simulink model "flatsat_data_send_2018"  (R2018b)
settings: Solver=VariableStepAuto  StartTime=0.0  StopTime=Inf  RelTol=1e-3
values from neighbouring files (symbols this model uses):
  bias_sun_detection = 50    [flatsat_data_send_init.m]
  magnitude_gyro = 250    [flatsat_data_send_init.m]
  magnitude_mag = 100    [flatsat_data_send_init.m]
  magnitude_phd = 100    [flatsat_data_send_init.m]
  magnitude_sun_angle = 60    [flatsat_data_send_init.m]
  magnitude_sun_detection = 50    [flatsat_data_send_init.m]
  t_receive_gyro = t_send_gyro    (= 0.04)    [flatsat_data_send_init.m]
  t_receive_sun = t_send_sun    (= 0.02)    [flatsat_data_send_init.m]
  t_send_gyro = 1/25    (= 0.04)    [flatsat_data_send_init.m]
  t_send_mag = 1/15    (= 0.0666666666667)    [flatsat_data_send_init.m]
  t_send_phd = 0.061    [flatsat_data_send_init.m]
  t_send_sun = 0.02    [flatsat_data_send_init.m]
undefined symbols (not defined in the file or in its folder): serial, t_receive
libraries: instrumentlib x12
settings Model: EnablePacing=on  Creator=Alex Zhen  LastModifiedBy=Alex Zhen
settings DataIOCC: ReturnWorkspaceOutputs=on

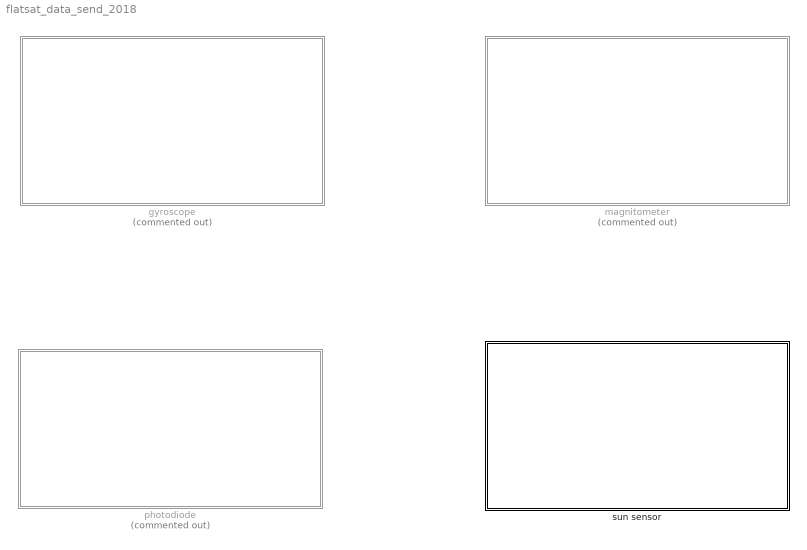
== system flatsat_data_send_2018 ==
  gyroscope : Subsystem  Commented=on
  magnitometer : Subsystem  Commented=on
  photodiode : Subsystem  Commented=on
  sun sensor : Subsystem

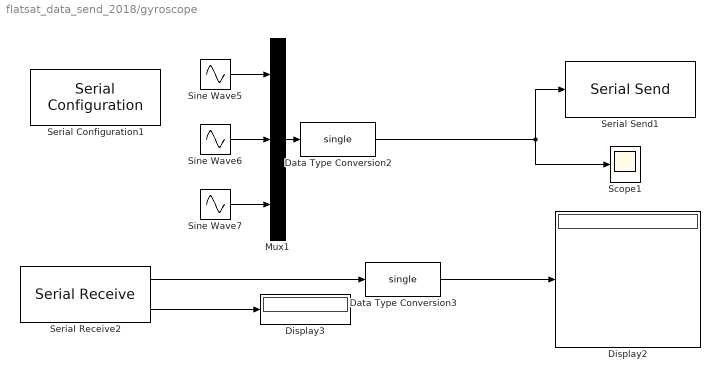
== system flatsat_data_send_2018/gyroscope ==
  Data Type Conversion2 : DataTypeConversion  OutDataTypeStr=single
  Data Type Conversion3 : DataTypeConversion  OutDataTypeStr=single
  Display2 : Display
  Display3 : Display
  Mux1 : Mux  Inputs=3
  Scope1 : Scope
  Serial Configuration1 : instrumentlib/Serial Configuration  Priority=-200000  ComPortMenu=COM5  ComPort=COM5  ObjConstructor=serial('COM5');  BaudRate=115200  DataBits=8  Parity=none  StopBits=1  FlowControl=none  Timeout=10  ByteOrder=LittleEndian
  Serial Receive2 : instrumentlib/Serial Receive  ComPortMenu=COM5  ComPort=COM5  ObjConstructor=serial('COM5');  Terminator=<none>  DataSize="[3  1]"  DataType=single  EnableBlockingMode=off  ActionDataUnavailable=Output last received value  CustomValue=0  SampleTime=t_receive_gyro
  Serial Send1 : instrumentlib/Serial Send  ComPortMenu=COM5  ComPort=COM5  ObjConstructor=serial('COM5');  Terminator=<none>  EnableBlockingMode=off
  Sine Wave5 : Sin  Amplitude=magnitude_gyro  Frequency=pi/5  SampleTime=t_send_gyro
  Sine Wave6 : Sin  Amplitude=magnitude_gyro  Frequency=pi/5  Phase=1  SampleTime=t_send_gyro
  Sine Wave7 : Sin  Amplitude=magnitude_gyro  Frequency=pi/5  Phase=2  SampleTime=t_send_gyro
  wires:
  Data Type Conversion2/1 -> Serial Send1/1, Scope1/1
  Data Type Conversion3/1 -> Display2/1
  Sine Wave5/1 -> Mux1/1
  Serial Receive2/1 -> Data Type Conversion3/1
  Sine Wave6/1 -> Mux1/2
  Sine Wave7/1 -> Mux1/3
  Mux1/1 -> Data Type Conversion2/1
  Serial Receive2/2 -> Display3/1

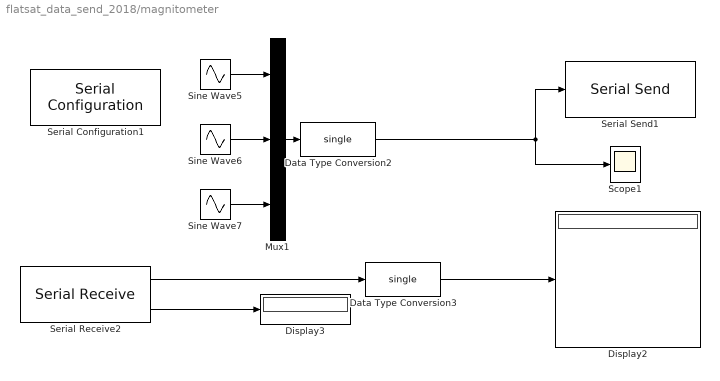
== system flatsat_data_send_2018/magnitometer ==
  Data Type Conversion2 : DataTypeConversion  OutDataTypeStr=single
  Data Type Conversion3 : DataTypeConversion  OutDataTypeStr=single
  Display2 : Display
  Display3 : Display
  Mux1 : Mux  Inputs=3
  Scope1 : Scope
  Serial Configuration1 : instrumentlib/Serial Configuration  Priority=-200000  ComPortMenu=COM5  ComPort=COM5  ObjConstructor=serial('COM5');  BaudRate=115200  DataBits=8  Parity=none  StopBits=1  FlowControl=none  Timeout=10  ByteOrder=LittleEndian
  Serial Receive2 : instrumentlib/Serial Receive  ComPortMenu=COM5  ComPort=COM5  ObjConstructor=serial('COM5');  Terminator=<none>  DataSize="[3  1]"  DataType=single  EnableBlockingMode=off  ActionDataUnavailable=Output last received value  CustomValue=0  SampleTime=t_receive_gyro
  Serial Send1 : instrumentlib/Serial Send  ComPortMenu=COM5  ComPort=COM5  ObjConstructor=serial('COM5');  Terminator=<none>  EnableBlockingMode=off
  Sine Wave5 : Sin  Amplitude=magnitude_mag  Frequency=pi/5  SampleTime=t_send_mag
  Sine Wave6 : Sin  Amplitude=magnitude_mag  Frequency=pi/5  Phase=1  SampleTime=t_send_mag
  Sine Wave7 : Sin  Amplitude=magnitude_mag  Frequency=pi/5  Phase=2  SampleTime=t_send_mag
  wires:
  Data Type Conversion2/1 -> Serial Send1/1, Scope1/1
  Data Type Conversion3/1 -> Display2/1
  Sine Wave5/1 -> Mux1/1
  Serial Receive2/1 -> Data Type Conversion3/1
  Sine Wave6/1 -> Mux1/2
  Sine Wave7/1 -> Mux1/3
  Mux1/1 -> Data Type Conversion2/1
  Serial Receive2/2 -> Display3/1

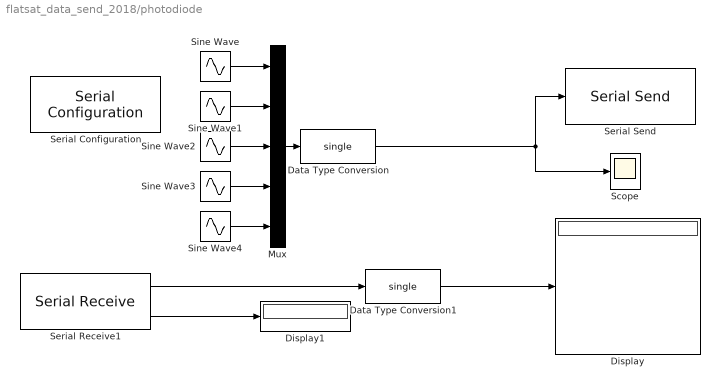
== system flatsat_data_send_2018/photodiode ==
  Data Type Conversion : DataTypeConversion  OutDataTypeStr=single
  Data Type Conversion1 : DataTypeConversion  OutDataTypeStr=single
  Display : Display
  Display1 : Display
  Mux : Mux  Inputs=5
  Scope : Scope
  Serial Configuration : instrumentlib/Serial Configuration  Priority=-200000  ComPortMenu=COM5  ComPort=COM5  ObjConstructor=serial('COM5');  BaudRate=115200  DataBits=8  Parity=none  StopBits=1  FlowControl=none  Timeout=10  ByteOrder=LittleEndian
  Serial Receive1 : instrumentlib/Serial Receive  ComPortMenu=COM5  ComPort=COM5  ObjConstructor=serial('COM5');  Terminator=<none>  DataSize="[5  1]"  DataType=single  EnableBlockingMode=off  ActionDataUnavailable=Output last received value  CustomValue=0  SampleTime=t_receive
  Serial Send : instrumentlib/Serial Send  ComPortMenu=COM5  ComPort=COM5  ObjConstructor=serial('COM5');  Terminator=<none>  EnableBlockingMode=off
  Sine Wave : Sin  Amplitude=magnitude_phd  Frequency=pi/5  SampleTime=t_send_phd
  Sine Wave1 : Sin  Amplitude=250  Frequency=pi/5  Phase=1  SampleTime=t_send_phd
  Sine Wave2 : Sin  Amplitude=magnitude_phd  Frequency=pi/5  Phase=2  SampleTime=t_send_phd
  Sine Wave3 : Sin  Amplitude=magnitude_phd  Frequency=pi/5  Phase=3  SampleTime=t_send_phd
  Sine Wave4 : Sin  Amplitude=magnitude_phd  Frequency=pi/5  Phase=4  SampleTime=t_send_phd
  wires:
  Sine Wave1/1 -> Mux/2
  Data Type Conversion/1 -> Serial Send/1, Scope/1
  Serial Receive1/2 -> Display1/1
  Data Type Conversion1/1 -> Display/1
  Sine Wave3/1 -> Mux/4
  Sine Wave2/1 -> Mux/3
  Serial Receive1/1 -> Data Type Conversion1/1
  Sine Wave/1 -> Mux/1
  Mux/1 -> Data Type Conversion/1
  Sine Wave4/1 -> Mux/5

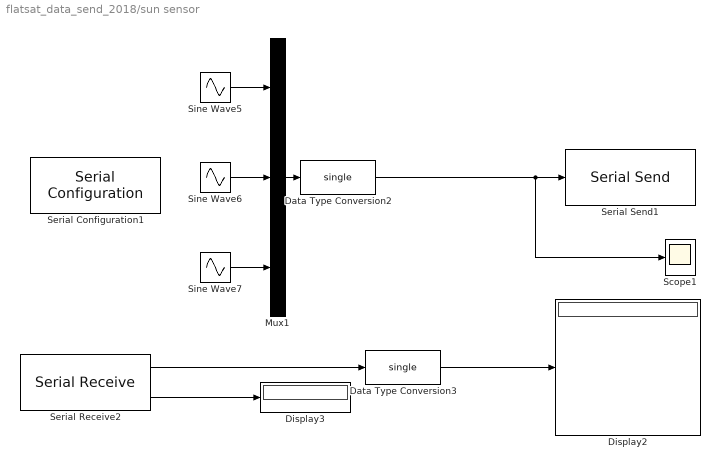
== system flatsat_data_send_2018/sun sensor ==
  Data Type Conversion2 : DataTypeConversion  OutDataTypeStr=single
  Data Type Conversion3 : DataTypeConversion  OutDataTypeStr=single
  Display2 : Display
  Display3 : Display
  Mux1 : Mux  Inputs=3
  Scope1 : Scope
  Serial Configuration1 : instrumentlib/Serial Configuration  Priority=-200000  ComPortMenu=COM9  ComPort=COM9  ObjConstructor=serial('COM9');  BaudRate=115200  DataBits=8  Parity=none  StopBits=1  FlowControl=none  Timeout=10  ByteOrder=LittleEndian
  Serial Receive2 : instrumentlib/Serial Receive  ComPortMenu=COM9  ComPort=COM9  ObjConstructor=serial('COM9');  Terminator=<none>  DataSize="[3  1]"  DataType=single  EnableBlockingMode=off  ActionDataUnavailable=Output last received value  CustomValue=0  SampleTime=t_receive_sun
  Serial Send1 : instrumentlib/Serial Send  ComPortMenu=COM9  ComPort=COM9  ObjConstructor=serial('COM9');  Terminator=<none>  EnableBlockingMode=off
  Sine Wave5 : Sin  Amplitude=magnitude_sun_angle  Frequency=pi/5  SampleTime=t_send_sun
  Sine Wave6 : Sin  Amplitude=magnitude_sun_angle  Frequency=pi/5  Phase=1  SampleTime=t_send_sun
  Sine Wave7 : Sin  Amplitude=magnitude_sun_detection  Bias=bias_sun_detection  Frequency=pi/5  Phase=2  SampleTime=t_send_sun
  wires:
  Data Type Conversion2/1 -> Scope1/1, Serial Send1/1
  Data Type Conversion3/1 -> Display2/1
  Sine Wave5/1 -> Mux1/1
  Serial Receive2/1 -> Data Type Conversion3/1
  Sine Wave6/1 -> Mux1/2
  Sine Wave7/1 -> Mux1/3
  Mux1/1 -> Data Type Conversion2/1
  Serial Receive2/2 -> Display3/1
